simulink model "SHIY2"  (Simulink 6.3)
settings: Solver=ode45  StartTime=0.0  StopTime=500  RelTol=1e-3
libraries: fuzblock x2
settings Model: LastModifiedBy=Administrator

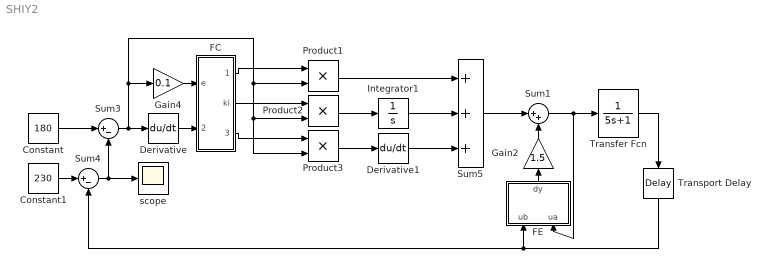
== system SHIY2 ==
  Constant : Constant  Value=180
  Constant1 : Constant  Value=230
  Derivative : Derivative
  Derivative1 : Derivative
  FC : Subsystem
  FE : Subsystem  Orientation=up
  Gain2 : Gain  Orientation=up  Gain=1.5
  Gain4 : Gain  Gain=0.1
  Integrator1 : Integrator
  Product1 : Product  RndMeth=Zero
  Product2 : Product  RndMeth=Zero
  Product3 : Product  RndMeth=Zero
  Sum1 : Sum  Inputs=|++
  Sum3 : Sum  Inputs=|+-
  Sum4 : Sum  Inputs=|+-
  Sum5 : Sum  Inputs=+++
  Transfer Fcn : TransferFcn  Denominator=[5 1]
  Transport Delay : TransportDelay  Orientation=down  DelayTime=10
  scope : Scope
      settings: TimeRange=200  YMin=180  YMax=180.6  SaveName=ScopeData3
  wires:
  Derivative/1 -> FC/2(de)
  Sum3/1 -> Derivative/1, Gain4/1, Product1/2, Product3/2, Product2/2
  Transfer Fcn/1 -> Transport Delay/1
  FE/1(dy) -> Gain2/1
  Constant/1 -> Sum3/1
  Constant1/1 -> Sum4/1
  Gain2/1 -> Sum1/2
  Sum1/1 -> Transfer Fcn/1, FE/2(ua)
  Gain4/1 -> FC/1(e)
  Product2/1 -> Integrator1/1
  Product3/1 -> Derivative1/1
  Sum5/1 -> Sum1/1
  Product1/1 -> Sum5/1
  Integrator1/1 -> Sum5/2
  FC/1(kp) -> Product1/1
  FC/2("ki ") -> Product2/1
  FC/3(kd) -> Product3/1
  Sum4/1 -> Sum3/2, scope/1
  Transport Delay/1 -> FE/1(ub), Sum4/2
  Derivative1/1 -> Sum5/3

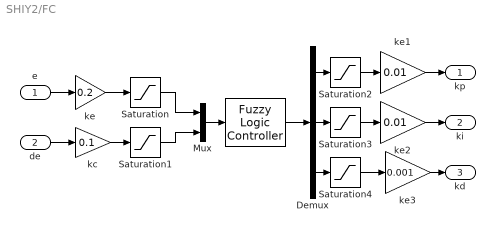
== system SHIY2/FC ==
  e : Inport
  de : Inport  Port=2
  " " : fuzblock/Fuzzy Logic  Controller  fis=fuzzyFC7
  Demux : Demux  Outputs=3
  Mux : Mux  Inputs=2
  Saturation{,1..4} (5 alike) : Saturate  UpperLimit=6  LowerLimit=-6
  kc : Gain  Gain=0.1
  ke : Gain  Gain=0.2
  ke1 : Gain  Gain=0.01
  ke2 : Gain  Gain=0.01
  ke3 : Gain  Gain=0.001
  kp : Outport
  "ki " : Outport  Port=2
  kd : Outport  Port=3
  wires:
  " "/1 -> Demux/1
  Saturation/1 -> Mux/1
  e/1 -> ke/1
  de/1 -> kc/1
  kc/1 -> Saturation1/1
  ke/1 -> Saturation/1
  Saturation1/1 -> Mux/2
  Mux/1 -> " "/1
  Demux/1 -> Saturation2/1
  Demux/2 -> Saturation3/1
  Demux/3 -> Saturation4/1
  Saturation2/1 -> ke1/1
  ke1/1 -> kp/1
  Saturation3/1 -> ke2/1
  ke2/1 -> "ki "/1
  Saturation4/1 -> ke3/1
  ke3/1 -> kd/1

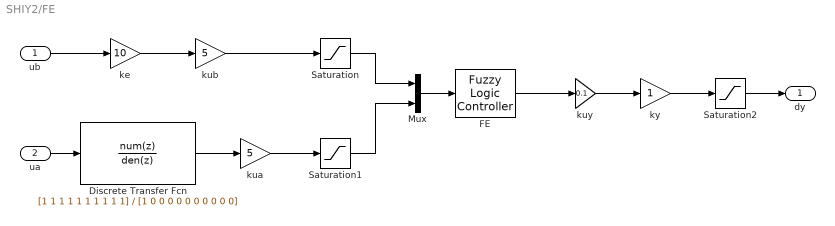
== system SHIY2/FE ==
  ub : Inport
  ua : Inport  Port=2
  Discrete Transfer Fcn : DiscreteTransferFcn  Numerator=[1 1 1 1 1 1 1 1 1 1]  Denominator=[1 0 0 0 0 0 0 0 0 0 0]
  FE : fuzblock/Fuzzy Logic  Controller  fis=fuzzyFE
  Mux : Mux  Inputs=2
  Saturation : Saturate  UpperLimit=6  LowerLimit=-6
  Saturation1 : Saturate  UpperLimit=6  LowerLimit=-6
  Saturation2 : Saturate  UpperLimit=6  LowerLimit=-6
  ke : Gain  Gain=10
  kua : Gain  Gain=5
  kub : Gain  Gain=5
  kuy : Gain  Gain=0.1
  ky : Gain
  dy : Outport
  wires:
  kuy/1 -> ky/1
  Discrete Transfer Fcn/1 -> kua/1
  kub/1 -> Saturation/1
  ub/1 -> ke/1
  ua/1 -> Discrete Transfer Fcn/1
  kua/1 -> Saturation1/1
  ke/1 -> kub/1
  Saturation/1 -> Mux/1
  Saturation1/1 -> Mux/2
  Mux/1 -> FE/1
  FE/1 -> kuy/1
  ky/1 -> Saturation2/1
  Saturation2/1 -> dy/1
